simulink library "ad_common"  (R2017a)
settings: Solver=VariableStepAuto  StartTime=0.0  StopTime=10.0  RelTol=1e-3
libraries: autodiff x5, ad_common x1
settings Model: Creator=eruffaldi  LastModifiedBy=eruffaldi

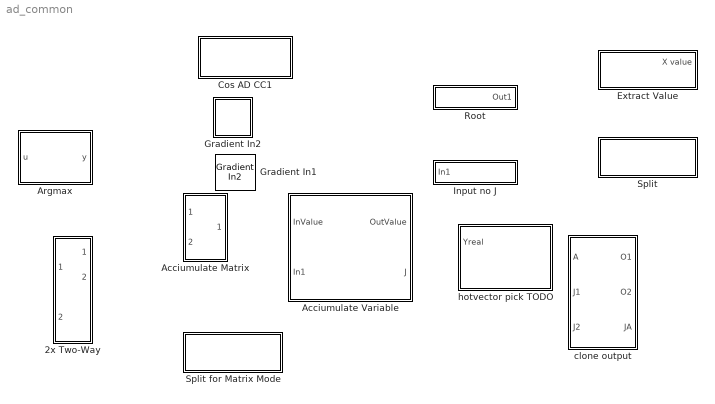
== system ad_common ==
  "2x Two-Way " : Subsystem
  Acciumulate Matrix : Subsystem  mask{Inputs=2}
      mask Callback Inputs:
      | x = gcb;
      | s = gcb;
      | asked = max(1,str2num(get_param(gcb,'Inputs')));
      | 
      | bcon = [x '/Matrix Concatenate'];
      | actual = str2num(get_param(bcon,'NumInputs'));
      | 
      | if asked == actual
      | else
      | bconL = bcon(length(x)+2:end);
      | 
      | if asked > actual
      |     set_param(bcon,'NumInputs',num2str(asked));
      |     bin1 = ([x '/In1']);
      |     bsh1 = ([x '/Reshape1']);
      |     bin1L = bin1(length(x)+2:end);
      |     bsh1L = bsh1(length(x)+2:end);
      |     for I=actual+1:asked
      |         bin = sprintf([x '/In%d'],I);
      |         bsh = sprintf([x '/Reshape%d'],I);
      |         binL = bin(length(x)+2:end);
      |         bshL = bsh(length(x)+2:end);
      |         % clone In and Reshape
      |         add_block(bin1,bin);
      |         add_block(bsh1,bsh);
      |         add_line(s,[binL '/1'],[bshL '/1']);
      |         add_line(s,[bshL '/1'],[bconL sprintf('/%d',I)]);
      |     end
      | else
      |     % remove
      |     for I=actual:-1:asked+1
      |         bin = sprintf([x '/In%d'],I);
      |         bsh = sprintf([x '/Reshape%d'],I);
      |         binL = bin(length(x)+2:end);
      |         bshL = bsh(length(x)+2:end);
      | 
      |         try
      |         delete_line(s,[binL '/1'],[bshL '/1']);
      |         catch me
      |         end
      |         try
      |         delete_line(s,[bshL '/1'],[bconL sprintf('/%d',I)]);
      |         catch me
      |         end
      |         try
      |         delete_block(bin);
      |         catch me
      |         end
      |         try
      |         delete_block(bsh);
      |         catch me
      |         end
      |     end
      |     set_param(bcon,'NumInputs',num2str(asked));
      | end
      | end
  Acciumulate Variable : Subsystem  mask{Inputs=1}
      mask Callback Inputs:
      | x = gcb;
      | s = gcb;
      | asked = max(1,str2num(get_param(gcb,'Inputs')));
      | 
      | bcon = [x '/Matrix Concatenate'];
      | actual = str2num(get_param(bcon,'NumInputs'));
      | 
      | if asked == actual
      | else
      | bconL = bcon(length(x)+2:end);
      | 
      | if asked > actual
      |     set_param(bcon,'NumInputs',num2str(asked));
      |     bin1 = ([x '/In1']);
      |     bsh1 = ([x '/Reshape1']);
      |     bin1L = bin1(length(x)+2:end);
      |     bsh1L = bsh1(length(x)+2:end);
      |     for I=actual+1:asked
      |         bin = sprintf([x '/In%d'],I);
      |         bsh = sprintf([x '/Reshape%d'],I);
      |         binL = bin(length(x)+2:end);
      |         bshL = bsh(length(x)+2:end);
      |         % clone In and Reshape
      |         add_block(bin1,bin);
      |         add_block(bsh1,bsh);
      |         add_line(s,[binL '/1'],[bshL '/1']);
      |         add_line(s,[bshL '/1'],[bconL sprintf('/%d',I)]);
      |     end
      | else
      |     % remove
      |     for I=actual:-1:asked+1
      |         bin = sprintf([x '/In%d'],I);
      |         bsh = sprintf([x '/Reshape%d'],I);
      |         binL = bin(length(x)+2:end);
      |         bshL = bsh(length(x)+2:end);
      | 
      |         try
      |         delete_line(s,[binL '/1'],[bshL '/1']);
      |         catch me
      |         end
      |         try
      |         delete_line(s,[bshL '/1'],[bconL sprintf('/%d',I)]);
      |         catch me
      |         end
      |         try
      |         delete_block(bin);
      |         catch me
      |         end
      |         try
      |         delete_block(bsh);
      |         catch me
      |         end
      |     end
      |     set_param(bcon,'NumInputs',num2str(asked));
      | end
      | end
  "Argmax " : MATLAB Function  TreatAsAtomicUnit=on  mask{dim=1}
      mask prompts: dim "Dimension"
  Cos AD CC1 : Subsystem  mask{gain=1.0}
      mask prompts: gain "Scalar Value"
      mask Display: disp(['Gain ' get_param(gcb,'gain')]);
  Extract Value : Subsystem
  Gradient In1 : ad_common/Gradient In2  SystemSampleTime=-1
  Gradient In2 : Subsystem
      mask Display: image('endroad.png');
  Input no J : Subsystem
      mask Display: disp('Input Only');
  Root : Subsystem
      mask Display: disp('Gradient Root');
  Split : Subsystem
  Split for Matrix Mode : Subsystem
  clone output : Subsystem
  hotvector pick TODO : Subsystem

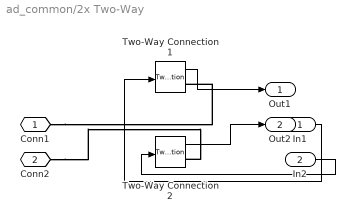
== system ad_common/2x Two-Way  ==
  In1 : Inport
  In2 : Inport  Port=2
  Two-Way Connection1 : TwoWayConnection
  Two-Way Connection2 : TwoWayConnection
  Conn1 : PMIOPort  Port=1  Side=Right
  Conn2 : PMIOPort  Port=2  Side=Right
  Out1 : Outport
  Out2 : Outport  Port=2
  wires:
  Two-Way Connection1/1 -> Out1/1
  In1/1 -> Two-Way Connection1/1
  Two-Way Connection2/1 -> Out2/1
  In2/1 -> Two-Way Connection2/1
  connections:
  Conn1/RConn1 -- Two-Way Connection1/RConn1
  Conn2/RConn1 -- Two-Way Connection2/RConn1

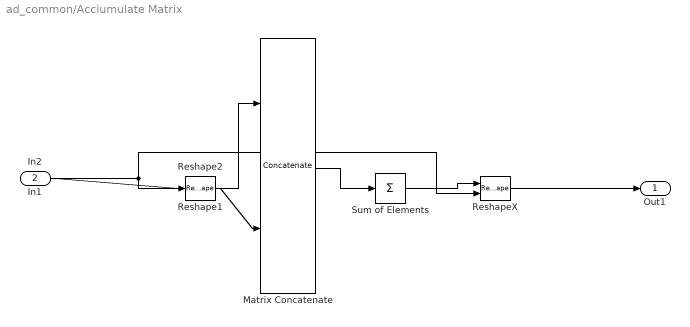
== system ad_common/Acciumulate Matrix ==
  In1 : Inport
  In2 : Inport  Port=2
  Matrix Concatenate : Concatenate  Mode=Multidimensional array  ConcatenateDimension=2
  Reshape1 : Reshape
  Reshape2 : Reshape
  ReshapeX : Reshape  OutputDimensionality=Derive from reference input port
  Sum of Elements : Sum  Inputs=+  CollapseMode=Specified dimension  CollapseDim=2
  Out1 : Outport
  wires:
  Sum of Elements/1 -> ReshapeX/1
  In1/1 -> ReshapeX/2, Reshape1/1
  Reshape1/1 -> Matrix Concatenate/1
  Matrix Concatenate/1 -> Sum of Elements/1
  ReshapeX/1 -> Out1/1
  In2/1 -> Reshape2/1
  Reshape2/1 -> Matrix Concatenate/2

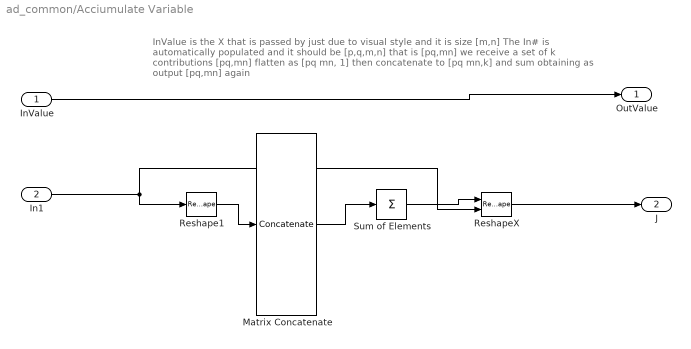
== system ad_common/Acciumulate Variable ==
  note: InValue is the X that is passed by just due to visual style and it is size [m,n]
      |
      | The In# is automatically populated and it should be [p,q,m,n] that is [pq,mn] we
      | receive a set of k contributions [pq,mn] flatten as [pq mn, 1] then concatenate to [pq mn,k]
      | and sum obtaining as output [pq,mn] again
  InValue : Inport
  In1 : Inport  Port=2
  Matrix Concatenate : Concatenate  NumInputs=1  Mode=Multidimensional array  ConcatenateDimension=2
  Reshape1 : Reshape
  ReshapeX : Reshape  OutputDimensionality=Derive from reference input port
  Sum of Elements : Sum  Inputs=+  CollapseMode=Specified dimension  CollapseDim=2
  OutValue : Outport
  J : Outport  Port=2
  wires:
  Sum of Elements/1 -> ReshapeX/1
  In1/1 -> ReshapeX/2, Reshape1/1
  Reshape1/1 -> Matrix Concatenate/1
  Matrix Concatenate/1 -> Sum of Elements/1
  ReshapeX/1 -> J/1
  InValue/1 -> OutValue/1

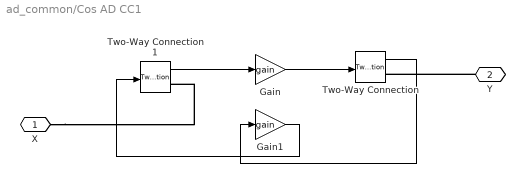
== system ad_common/Cos AD CC1 ==
  Gain : Gain  Gain=gain
  Gain1 : Gain  Gain=gain
  Two-Way Connection : TwoWayConnection
  Two-Way Connection1 : TwoWayConnection
  X : PMIOPort  Port=1  Side=Left
  Y : PMIOPort  Port=2  Side=Right
  wires:
  Two-Way Connection/1 -> Gain1/1
  Gain/1 -> Two-Way Connection/1
  Two-Way Connection1/1 -> Gain/1
  Gain1/1 -> Two-Way Connection1/1
  connections:
  X/RConn1 -- Two-Way Connection1/RConn1
  Y/RConn1 -- Two-Way Connection/RConn1

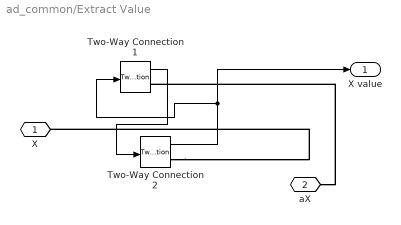
== system ad_common/Extract Value ==
  Two-Way Connection1 : TwoWayConnection
  Two-Way Connection2 : TwoWayConnection
  X : PMIOPort  Port=1  Side=Left
  aX : PMIOPort  Port=2  Side=Right
  X value : Outport
  wires:
  Two-Way Connection2/1 -> Two-Way Connection1/1, X value/1
  Two-Way Connection1/1 -> Two-Way Connection2/1
  connections:
  aX/RConn1 -- Two-Way Connection1/RConn1
  Two-Way Connection2/RConn1 -- X/RConn1

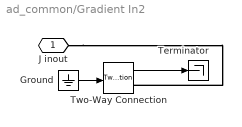
== system ad_common/Gradient In2 ==
  Ground : Ground
  Terminator : Terminator
  Two-Way Connection : TwoWayConnection
  J inout : PMIOPort  Port=1  Side=Right
  wires:
  Ground/1 -> Two-Way Connection/1
  Two-Way Connection/1 -> Terminator/1
  connections:
  J inout/RConn1 -- Two-Way Connection/RConn1

== system ad_common/Input no J ==
  In1 : Inport
  Terminator : Terminator
  Two-Way Connection1 : TwoWayConnection
  Conn1 : PMIOPort  Port=1  Side=Right
  wires:
  Two-Way Connection1/1 -> Terminator/1
  In1/1 -> Two-Way Connection1/1
  connections:
  Conn1/RConn1 -- Two-Way Connection1/RConn1

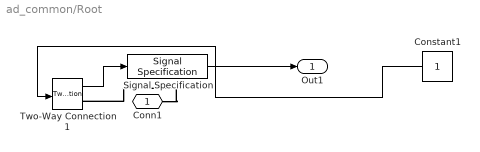
== system ad_common/Root ==
  Constant1 : Constant
  Signal Specification : SignalSpecification  Dimensions=1
  Two-Way Connection1 : TwoWayConnection
  Conn1 : PMIOPort  Port=1  Side=Left
  Out1 : Outport
  wires:
  Constant1/1 -> Two-Way Connection1/1
  Two-Way Connection1/1 -> Signal Specification/1
  Signal Specification/1 -> Out1/1
  connections:
  Conn1/RConn1 -- Two-Way Connection1/RConn1

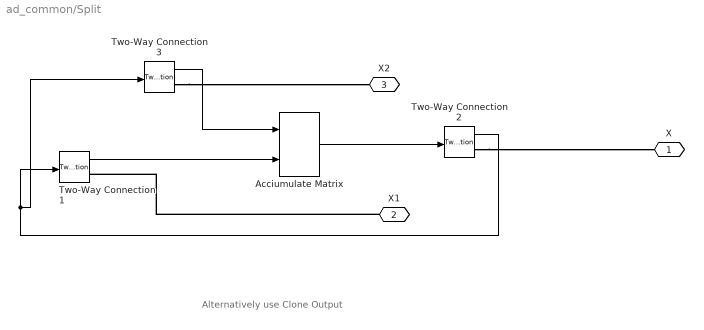
== system ad_common/Split ==
  note: Alternatively use Clone Output
  Acciumulate Matrix : autodiff/Common/Acciumulate Matrix  Inputs=2
      settings: SourceProductName=AutoDiff
  Two-Way Connection1 : TwoWayConnection
  Two-Way Connection2 : TwoWayConnection
  Two-Way Connection3 : TwoWayConnection
  X : PMIOPort  Port=1  Side=Left
  X1 : PMIOPort  Port=2  Side=Right
  X2 : PMIOPort  Port=3  Side=Right
  wires:
  Two-Way Connection2/1 -> Two-Way Connection3/1, Two-Way Connection1/1
  Two-Way Connection3/1 -> Acciumulate Matrix/1
  Two-Way Connection1/1 -> Acciumulate Matrix/2
  Acciumulate Matrix/1 -> Two-Way Connection2/1
  connections:
  Two-Way Connection2/RConn1 -- X/RConn1
  X1/RConn1 -- Two-Way Connection1/RConn1
  Two-Way Connection3/RConn1 -- X2/RConn1

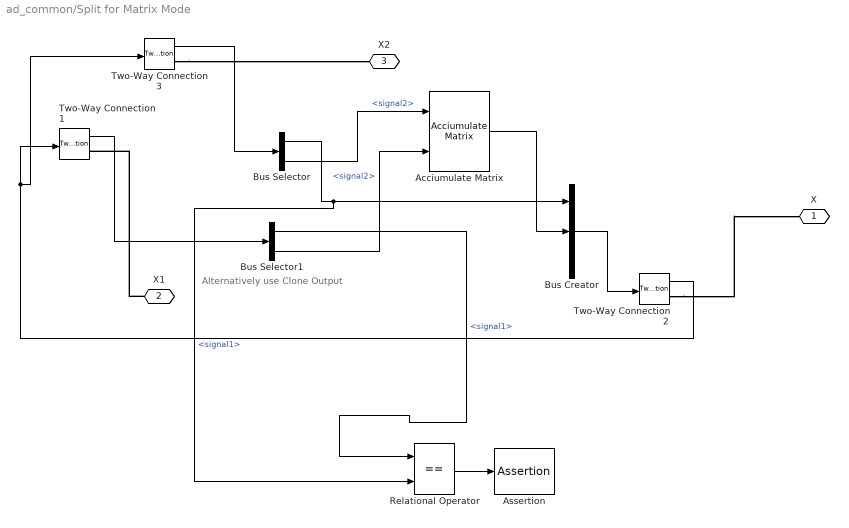
== system ad_common/Split for Matrix Mode ==
  note: Alternatively use Clone Output
  Acciumulate Matrix : autodiff/Common/Acciumulate Matrix  Inputs=2
      settings: SourceProductName=AutoDiff
  Assertion : Assertion
  Bus Creator : BusCreator  Inputs=3
  Bus Selector : BusSelector  OutputSignals=signal1,signal2
  Bus Selector1 : BusSelector  OutputSignals=signal1,signal2
  Relational Operator : RelationalOperator  Operator===  OutDataTypeStr=boolean  RndMeth=Simplest
  Two-Way Connection1 : TwoWayConnection
  Two-Way Connection2 : TwoWayConnection
  Two-Way Connection3 : TwoWayConnection
  X : PMIOPort  Port=1  Side=Left
  X1 : PMIOPort  Port=2  Side=Right
  X2 : PMIOPort  Port=3  Side=Right
  wires:
  Two-Way Connection2/1 -> Two-Way Connection1/1, Two-Way Connection3/1
  Bus Creator/1 -> Two-Way Connection2/1
  Two-Way Connection3/1 -> Bus Selector/1
  Acciumulate Matrix/1 -> Bus Creator/2
  Two-Way Connection1/1 -> Bus Selector1/1
  Bus Selector/2 -> Acciumulate Matrix/1  "<signal2>"
  Bus Selector1/2 -> Acciumulate Matrix/2  "<signal2>"
  Bus Selector/1 -> Relational Operator/2, Bus Creator/1  "<signal1>"
  Bus Selector1/1 -> Relational Operator/1  "<signal1>"
  Relational Operator/1 -> Assertion/1
  connections:
  Two-Way Connection3/RConn1 -- X2/RConn1
  X1/RConn1 -- Two-Way Connection1/RConn1
  Two-Way Connection2/RConn1 -- X/RConn1

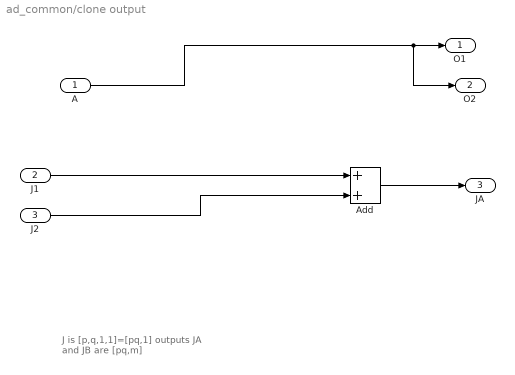
== system ad_common/clone output ==
  note: J is [p,q,1,1]=[pq,1]
      | outputs JA and JB are [pq,m]
  A : Inport
  J1 : Inport  Port=2
  "J2 " : Inport  Port=3
  Add : Sum
  O1 : Outport
  O2 : Outport  Port=2
  JA : Outport  Port=3
  wires:
  J1/1 -> Add/1
  Add/1 -> JA/1
  A/1 -> O2/1, O1/1
  "J2 "/1 -> Add/2

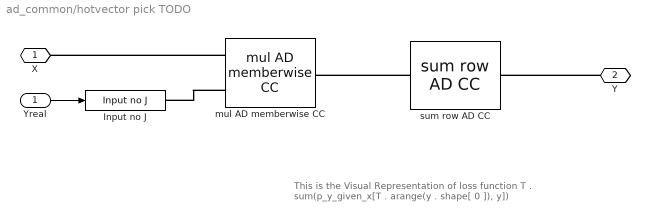
== system ad_common/hotvector pick TODO ==
  note: This is the Visual Representation of loss function
      |
      | T . sum(p_y_given_x[T . arange(y . shape[ 0 ]), y])
  Yreal : Inport
  Input no J : autodiff/Input no J  SystemSampleTime=-1
      settings: SourceProductName=AutoDiff
  mul AD memberwise CC : autodiff/mul AD memberwise CC
      settings: SourceProductName=AutoDiff
  sum row AD CC : autodiff/sum row AD CC  SystemSampleTime=-1
      settings: SourceProductName=AutoDiff
  X : PMIOPort  Port=1  Side=Left
  Y : PMIOPort  Port=2  Side=Right
  wires:
  Yreal/1 -> Input no J/1
  connections:
  mul AD memberwise CC/LConn1 -- X/RConn1
  Y/RConn1 -- sum row AD CC/RConn1
  mul AD memberwise CC/LConn2 -- Input no J/RConn1
  sum row AD CC/LConn1 -- mul AD memberwise CC/RConn1

== matlab function ad_common/Argmax  ==
  data: u input; y output double size=1; dim parameter size=1
function y = fcn(u, dim)
y = 0;
[~,y] = max(u,[],dim);
